simulink model "SC_Lab2_Variant3"  (R2025b)
settings: Solver=ode45  StartTime=0.0  StopTime=1  RelTol=1e-3
settings Model: Creator=m  LastModifiedBy=m
settings DataIOCC: SaveFormat=StructureWithTime

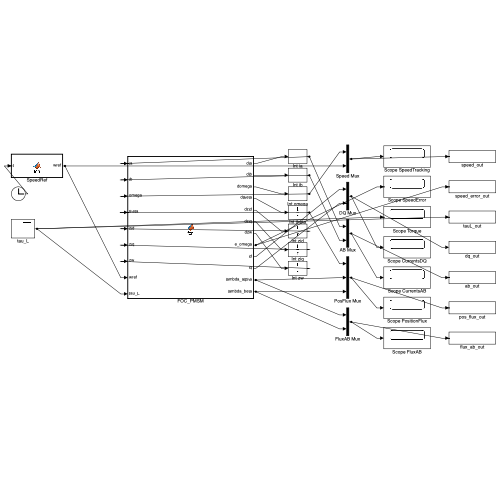
[thumbnail: Simulink's stored preview of the top-level diagram]
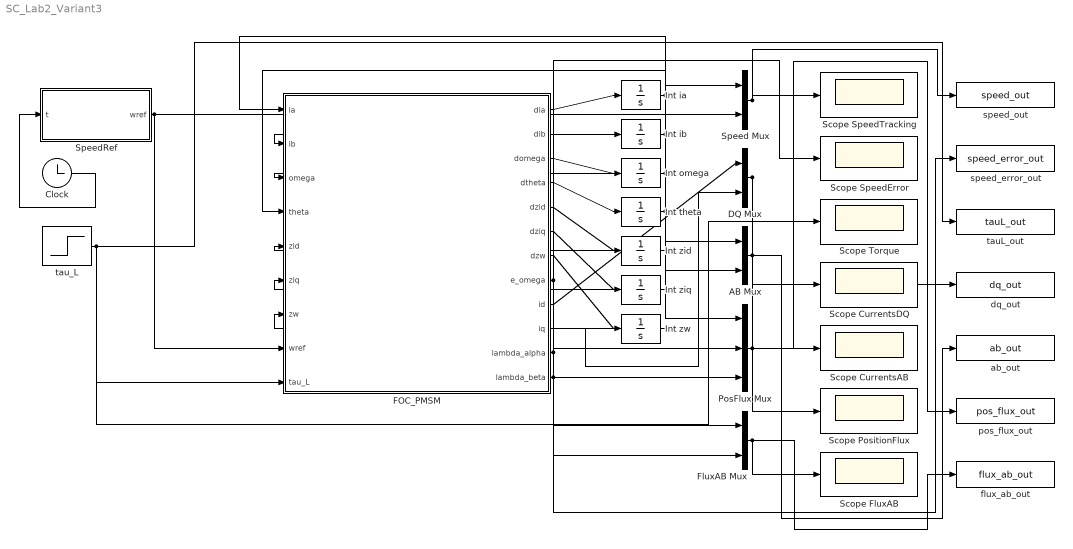
== system SC_Lab2_Variant3 ==
  AB Mux : Mux  Inputs=2
  Clock : Clock
  DQ Mux : Mux  Inputs=2
  FOC_PMSM : MATLAB Function  TreatAsAtomicUnit=on
  FluxAB Mux : Mux  Inputs=2
  Int ia : Integrator
  Int ib : Integrator
  Int omega : Integrator
  Int theta : Integrator
  Int zid : Integrator
  Int ziq : Integrator
  Int zw : Integrator
  PosFlux Mux : Mux  Inputs=3
  Scope CurrentsAB : Scope
  Scope CurrentsDQ : Scope
  Scope FluxAB : Scope
  Scope PositionFlux : Scope
  Scope SpeedError : Scope
  Scope SpeedTracking : Scope
  Scope Torque : Scope
  Speed Mux : Mux  Inputs=2
  SpeedRef : MATLAB Function  TreatAsAtomicUnit=on
  ab_out : ToWorkspace  VariableName=ab_out  SaveFormat=Structure With Time  SampleTime=-1
  dq_out : ToWorkspace  VariableName=dq_out  SaveFormat=Structure With Time  SampleTime=-1
  flux_ab_out : ToWorkspace  VariableName=flux_ab_out  SaveFormat=Structure With Time  SampleTime=-1
  pos_flux_out : ToWorkspace  VariableName=pos_flux_out  SaveFormat=Structure With Time  SampleTime=-1
  speed_error_out : ToWorkspace  VariableName=speed_error_out  SaveFormat=Structure With Time  SampleTime=-1
  speed_out : ToWorkspace  VariableName=speed_out  SaveFormat=Structure With Time  SampleTime=-1
  tauL_out : ToWorkspace  VariableName=tauL_out  SaveFormat=Structure With Time  SampleTime=-1
  tau_L : Step  Time=0.5  After=0.35  SampleTime=0
  wires:
  Clock/1 -> SpeedRef/1(t)
  SpeedRef/1(wref) -> FOC_PMSM/8(wref), Speed Mux/2
  tau_L/1 -> FOC_PMSM/9(tau_L), Scope Torque/1, tauL_out/1
  Int ia/1 -> FOC_PMSM/1(ia), AB Mux/1
  Int ib/1 -> FOC_PMSM/2(ib), AB Mux/2
  Int omega/1 -> FOC_PMSM/3(omega), Speed Mux/1
  Int theta/1 -> FOC_PMSM/4(theta), PosFlux Mux/1
  Int zid/1 -> FOC_PMSM/5(zid)
  Int ziq/1 -> FOC_PMSM/6(ziq)
  Int zw/1 -> FOC_PMSM/7(zw)
  FOC_PMSM/1(dia) -> Int ia/1
  FOC_PMSM/2(dib) -> Int ib/1
  FOC_PMSM/3(domega) -> Int omega/1
  FOC_PMSM/4(dtheta) -> Int theta/1
  FOC_PMSM/5(dzid) -> Int zid/1
  FOC_PMSM/6(dziq) -> Int ziq/1
  FOC_PMSM/7(dzw) -> Int zw/1
  Speed Mux/1 -> Scope SpeedTracking/1, speed_out/1
  FOC_PMSM/8(e_omega) -> Scope SpeedError/1, speed_error_out/1
  FOC_PMSM/9(id) -> DQ Mux/1
  FOC_PMSM/10(iq) -> DQ Mux/2
  DQ Mux/1 -> Scope CurrentsDQ/1, dq_out/1
  AB Mux/1 -> Scope CurrentsAB/1, ab_out/1
  FOC_PMSM/11(lambda_alpha) -> PosFlux Mux/2, FluxAB Mux/1
  FOC_PMSM/12(lambda_beta) -> PosFlux Mux/3, FluxAB Mux/2
  PosFlux Mux/1 -> Scope PositionFlux/1, pos_flux_out/1
  FluxAB Mux/1 -> Scope FluxAB/1, flux_ab_out/1

== matlab function SC_Lab2_Variant3/FOC_PMSM ==
  data: ia input; dia output; ib input; omega input; theta input; zid input; ziq input; zw input; wref input; tau_L input; dib output; domega output; dtheta output; dzid output; dziq output; dzw output; e_omega output; id output; iq output; lambda_alpha output; lambda_beta output
function [dia, dib, domega, dtheta, dzid, dziq, dzw, e_omega, id, iq, lambda_alpha, lambda_beta] = fcn(ia, ib, omega, theta, zid, ziq, zw, wref, tau_L)
                                                                                                                                                      L = 0.033;                                                                                                                                             
                                                                                                                                                      R = 5.3;                                                                                                                                               
                                                                                                                                                      Jm = 0.0006;                                                                                                                                           
                                                                                                                                                      np = 5;                                                                                                                                                
                                                                                                                                                      lambda_m = 0.16;                                                                                                                                       
                                                                                                                                                      B = 0;                                                                                                                                                 
                                                                                                                                                      kp_i = 18;                                                                                                                                             
                                                                                                                                                      ki_i = 1400;                                                                                                                                           
                                                                                                                                                      kp_w = 0.36;                                                                                                                                           
                                                                                                                                                      ki_w = 18;                                                                                                                                             
                                                                                                                                                      iq_limit = 25;                                                                                                                                         
                                                                                                                                                      v_limit = 120;                                                                                                                                         
                                                                                                                                                      theta_e = np * theta;                                                                                                                                  
                                                                                                                                                      c = cos(theta_e);                                                                                                                                      
                                                                                                                                                      s = sin(theta_e);                                                                                                                                      
                                                                                                                                                      id = c*ia + s*ib;                                                                                                                                      
                                                                                                                                                      iq = -s*ia + c*ib;                                                                                                                                     
                                                                                                                                                      e_omega = wref - omega;                                                                                                                                
                                                                                                                                                      iq_ref = kp_w*e_omega + ki_w*zw;                                                                                                                       
                                                                                                                                                      if iq_ref > iq_limit                                                                                                                                   
                                                                                                                                                          iq_ref = iq_limit;                                                                                                                                 
                                                                                                                                                      elseif iq_ref < -iq_limit                                                                                                                              
                                                                                                                                                          iq_ref = -iq_limit;                                                                                                                                
                                                                                                                                                      end                                                                                                                                                    
                                                                                                                                                      id_ref = 0;                                                                                                                                            
                                                                                                                                                      e_id = id_ref - id;                                                                                                                                    
                                                                                                                                                      e_iq = iq_ref - iq;                                                                                                                                    
                                                                                                                                                      vd = kp_i*e_id + ki_i*zid - np*omega*L*iq;                                                                                                             
                                                                                                                                                      vq = kp_i*e_iq + ki_i*ziq + np*omega*(L*id + lambda_m);                                                                                                
                                                                                                                                                      va = c*vd - s*vq;                                                                                                                                      
                                                                                                                                                      vb = s*vd + c*vq;                                                                                                                                      
                                                                                                                                                      vnorm = sqrt(va*va + vb*vb);                                                                                                                           
                                                                                                                                                      if vnorm > v_limit                                                                                                                                     
                                                                                                                                                          scale = v_limit / vnorm;                                                                                                                           
                                                                                                                                                          va = va * scale;                                                                                                                                   
                                                                                                                                                          vb = vb * scale;                                                                                                                                   
                                                                                                                                                      end                                                                                                                                                    
                                                                                                                                                      dia = (-R*ia + va + lambda_m*np*omega*s) / L;                                                                                                          
                                                                                                                                                      dib = (-R*ib + vb - lambda_m*np*omega*c) / L;                                                                                                          
                                                                                                                                                      tau_e = np * lambda_m * (-ia*s + ib*c);                                                                                                                
                                                                                                                                                      domega = (-B*omega + tau_e - tau_L) / Jm;                                                                                                              
                                                                                                                                                      dtheta = omega;                                                                                                                                        
                                                                                                                                                      dzid = e_id;                                                                                                                                           
                                                                                                                                                      dziq = e_iq;                                                                                                                                           
                                                                                                                                                      dzw = e_omega;                                                                                                                                         
                                                                                                                                                      lambda_alpha = L*ia + lambda_m*c;                                                                                                                      
                                                                                                                                                      lambda_beta = L*ib + lambda_m*s;

== matlab function SC_Lab2_Variant3/SpeedRef ==
  data: t input; wref output
function wref = fcn(t)
                     if t < 0.2            
                         wref = 530*t;     
                     else                  
                         wref = 106;       
                     end
